simulink model "Xe_Model_Redo_June_26"  (R2018a)
settings: Solver=VariableStepAuto  StartTime=0.0  StopTime=5E5+96*60*60  RelTol=1e-3
values from neighbouring files (symbols this model uses):
  A_pipe = pi*r_pipe^2    (= 0.0126676869774)    [Startup_Script.m]
  alpha_FS = 0.517E-16    (= 5.17e-17)    [Startup_Script.m]
  alpha_G_R1 = 0.334E-17    (= 3.34e-18)    [Startup_Script.m]
  alpha_G_R2 = 0.699E-17    (= 6.99e-18)    [Startup_Script.m]
  alpha_G_R3 = 0.669E-17    (= 6.69e-18)    [Startup_Script.m]
  alpha_G_R4 = 0.791E-18    (= 7.91e-19)    [Startup_Script.m]
  D_g = 2.37E-9    (= 2.37e-09)    [Startup_Script.m]
  epsilon = 0.1    [Startup_Script.m]
  eta_b = 1E-4    (= 0.0001)    [Startup_Script.m]
  eta_fs = 1.2E-4    (= 0.00012)    [Startup_Script.m]
  f_cv = 0.004    [Startup_Script.m]
  FS_Mu_A = 4340    [Startup_Script.m]
  FS_Mu_K = 0.084    [Startup_Script.m]
  FS_Mu_MSRE = 0.007027    [Startup_Script.m]
  FS_rho_A = 3.628    [Startup_Script.m]
  FS_rho_B = 0.00066    [Startup_Script.m]
  FS_rho_MSRE = 2082    [Startup_Script.m]
  gamma_i = 0.0293524    [Startup_Script.m]
  gamma_te = 0.0322482    [Startup_Script.m]
  gamma_xe = 0.00257324    [Startup_Script.m]
  h_fc = 1.6    [Startup_Script.m]
  H_Xe_a = 5.713e-13    [Startup_Script.m]
  H_Xe_b = -7.937e-10    [Startup_Script.m]
  H_Xe_c = 2.809e-07    [Startup_Script.m]
  HX_r_Tube = ((0.5-0.042)/2)*2.54E-2    (= 0.0058166)    [Startup_Script.m]
  HX_XS = HX_N_Tubes*(pi*HX_r_Tube^2)    (= 0.0168999490356)    [Startup_Script.m]
  k_b = 1.3806E-23    (= 1.3806e-23)    [Startup_Script.m]
  lambda_i = 2.9306070546251702E-5    (= 2.93060705463e-05)    [Startup_Script.m]
  lambda_te = 0.036481430555786593    (= 0.0364814305558)    [Startup_Script.m]
  lambda_xe = 2.0924e-05    [Startup_Script.m]
  N_FC_R1 = 12    [Startup_Script.m]
  N_FC_R2 = 940    [Startup_Script.m]
  N_FC_R3 = 108    [Startup_Script.m]
  N_FC_R4 = 78    [Startup_Script.m]
  P_pump = 35420    [Startup_Script.m]
  phi0 = 3.98E+17    (= 3.98e+17)    [Startup_Script.m]
  phi_G_R_1 = mean(interp1(phi_G_R,phi_G_phi, linspace(0,r_g_r1)))    [Startup_Script.m]
  phi_G_R_2 = mean(interp1(phi_G_R,phi_G_phi, linspace(r_g_r1,r_g_r2)))    [Startup_Script.m]
  phi_G_R_3 = mean(interp1(phi_G_R,phi_G_phi, linspace(r_g_r2,r_g_r3)))    [Startup_Script.m]
  phi_G_R_4 = mean(interp1(phi_G_R,phi_G_phi, linspace(r_g_r3,r_g_r4)))    [Startup_Script.m]
  Q_strpr = 0.003155    [Startup_Script.m]
  Q_tot = 0.07571    [Startup_Script.m]
  r_b = 0.000254    [Startup_Script.m]
  r_fc = 0.79e-2    (= 0.0079)    [Startup_Script.m]
  r_pipe = (5E-2*2.54)/2    (= 0.0635)    [Startup_Script.m]
  r_xe = 2.16E-10    (= 2.16e-10)    [Startup_Script.m]
  Re_CA = 25800    [Startup_Script.m]
  Re_LH = 1E4    (= 10000)    [Startup_Script.m]
  Re_UH = 1E4    (= 10000)    [Startup_Script.m]
  sig_a_xe = 1.18E-22    (= 1.18e-22)    [Startup_Script.m]
  Sig_f = 0.15    [Startup_Script.m]
  T_CA_0 = T_INLET    (= 907.594444444)    [Startup_Script.m]
  T_FP_0 = T_OUTLET    (= 935.372222222)    [Startup_Script.m]
  T_FS_R_1_0 = mean(interp1(R_fs_m,T_fs_K, linspace(0,r_g_r1)))    [Startup_Script.m]
  T_FS_R_2_0 = mean(interp1(R_fs_m,T_fs_K, linspace(r_g_r1,r_g_r2)))    [Startup_Script.m]
  T_FS_R_3_0 = mean(interp1(R_fs_m,T_fs_K, linspace(r_g_r2,r_g_r3)))    [Startup_Script.m]
  T_FS_R_4_0 = mean(interp1(R_fs_m,T_fs_K, linspace(r_g_r3,r_g_r4)))    [Startup_Script.m]
  T_G_R_1_0 = mean(interp1(R_gr_m,T_gr_K, linspace(0,r_g_r1)))    [Startup_Script.m]
  T_HX_0 = 0.5*(T_OUTLET + T_INLET)    (= 921.483333333)    [Startup_Script.m]
  T_LH_0 = T_INLET    (= 907.594444444)    [Startup_Script.m]
  T_Mes = 928.15    [Startup_Script.m]
  T_P100_0 = T_OUTLET    (= 935.372222222)    [Startup_Script.m]
  T_P101_0 = T_OUTLET    (= 935.372222222)    [Startup_Script.m]
  T_P102_0 = T_INLET    (= 907.594444444)    [Startup_Script.m]
  T_Salt_0 = 900    [Startup_Script.m]
  T_UH_0 = T_OUTLET    (= 935.372222222)    [Startup_Script.m]
  U_FC_R1 = 0.607    [Startup_Script.m]
  U_FC_R2 = 0.183    [Startup_Script.m]
  U_FC_R3 = 0.454    [Startup_Script.m]
  U_FC_R4 = 0.250    (= 0.25)    [Startup_Script.m]
  V_CA_0 = 9.7*cubed_foot_to_cubed_meter    (= 0.274673445)    [Startup_Script.m]
  V_FP_0 = (0.9+3.2)*cubed_foot_to_cubed_meter    (= 0.116099085)    [Startup_Script.m]
  V_HX_0 = 6.1*cubed_foot_to_cubed_meter    (= 0.172732785)    [Startup_Script.m]
  V_LH_0 = 10.0*cubed_foot_to_cubed_meter    (= 0.2831685)    [Startup_Script.m]
  V_P100_0 = 2.1*cubed_foot_to_cubed_meter    (= 0.059465385)    [Startup_Script.m]
  V_P101_0 = 0.8*cubed_foot_to_cubed_meter    (= 0.02265348)    [Startup_Script.m]
  V_P102_0 = 2.2*cubed_foot_to_cubed_meter    (= 0.06229707)    [Startup_Script.m]
  V_R1_0 = V_Core_FS_0 *N_FC_R1/N_FC_tot    (= 0.00753107712766)    [Startup_Script.m]
  V_R2_0 = V_Core_FS_0 *N_FC_R2/N_FC_tot    (= 0.589934375)    [Startup_Script.m]
  V_R3_0 = V_Core_FS_0 *N_FC_R3/N_FC_tot    (= 0.0677796941489)    [Startup_Script.m]
  V_R4_0 = V_Core_FS_0 *N_FC_R4/N_FC_tot    (= 0.0489520013298)    [Startup_Script.m]
  V_UH_0 = 10.5*cubed_foot_to_cubed_meter    (= 0.297326925)    [Startup_Script.m]
undefined symbols (not defined in the file or in its folder): magnitude, V_CA, V_HX, V_P2, V_P3, V_R1, V_R2, V_R3, V_R4, V_UH
libraries: simulink x4, dspindex x4, dspstat3 x4, SignalEditorBlockLib x2
(part 5 of 11)

== system Xe_Model_Redo_June_26/Graphite /Graphite Region 4/Graphite Stringer/HMat ==
  H_Mat : Inport
  T : Inport  Port=2
  k_m_g : Inport  Port=3
  rGhost : Inport  Port=4
  Calc H_Xe : Subsystem
  H_Gain : Product  Inputs=****//
  mul : Product
  Out1 : Outport
  wires:
  H_Mat/1 -> mul/1
  mul/1 -> Out1/1
  H_Gain/1 -> mul/2
  rGhost/1 -> H_Gain/6
  Calc H_Xe/1(H_Xe [m^-3 Pa^-1]) -> H_Gain/1
  T/1 -> Calc H_Xe/1(T_Salt [K]), H_Gain/3
  k_m_g/1 -> H_Gain/4
  [epsilon] -> H_Gain/5
  [R_gas] -> H_Gain/2

== system Xe_Model_Redo_June_26/Bubbles/Bubble Mass Transfer/Bubble Total KMA/HX KMA/CA  CV Area ==
  Node Vol. : Inport
  Node T : Inport  Port=2
  CV Vol to Mass Transfer Area1 : Subsystem
  Calc CV Vol W Temp : Subsystem
  A : Outport
  wires:
  CV Vol to Mass Transfer Area1/1(A) -> A/1
  Node T/1 -> Calc CV Vol W Temp/2(T)
  Node Vol./1 -> Calc CV Vol W Temp/1(Vol. Gas)
  Calc CV Vol W Temp/1(V Gas) -> CV Vol to Mass Transfer Area1/1(V)

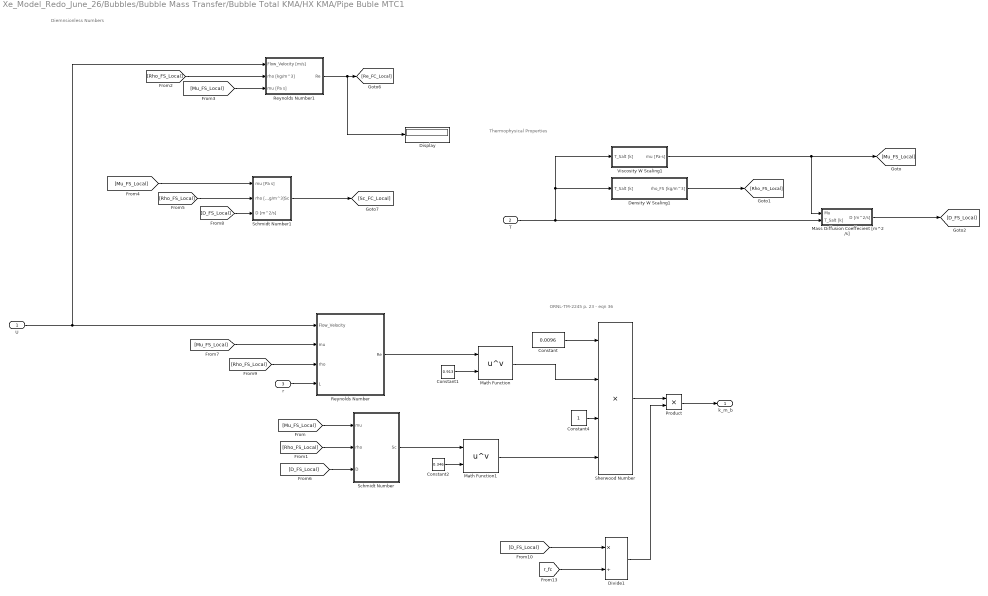
== system Xe_Model_Redo_June_26/Bubbles/Bubble Mass Transfer/Bubble Total KMA/HX KMA/Pipe Buble MTC1 ==
  note: ORNL-TM-2245 p. 23 - eqn 36
  note: Diemnsionless Numbers
  note: Thermophysical Properties
  U : Inport
  T : Inport  Port=2
  r : Inport  Port=3
  Constant : Constant  Value=0.0096
  Constant1 : Constant  Value=0.913
  Constant2 : Constant  Value=0.346
  Constant4 : Constant
  Density W Scaling1 : Subsystem
  Display : Display
  Divide1 : Product  Inputs=*/
  Mass Diffusion Coeffecient [m^2 /s] : Subsystem
  Math Function : Math  Operator=pow  SaturateOnIntegerOverflow=on
  Math Function1 : Math  Operator=pow  SaturateOnIntegerOverflow=on
  Product : Product
  Reynolds Number : Subsystem
  Reynolds Number1 : Subsystem
  Schmidt Number : Subsystem
  Schmidt Number1 : Subsystem
  Sherwood Number : Product  Inputs=4
  Viscosity W Scaling1 : Subsystem
  k_m_b : Outport
  wires:
  Constant1/1 -> Math Function/2
  [r_fc] -> Divide1/2
  Constant2/1 -> Math Function1/2
  [D_FS_Local] -> Divide1/1
  Constant4/1 -> Sherwood Number/3
  Constant/1 -> Sherwood Number/1
  Divide1/1 -> Product/2
  Math Function1/1 -> Sherwood Number/4
  Schmidt Number/1(Sc) -> Math Function1/1
  Math Function/1 -> Sherwood Number/2
  Sherwood Number/1 -> Product/1
  Product/1 -> k_m_b/1
  Reynolds Number/1(Re) -> Math Function/1
  Schmidt Number1/1(Sc) -> [Sc_FC_Local]
  Reynolds Number1/1(Re) -> Display/1, [Re_FC_Local]
  U/1 -> Reynolds Number1/1(Flow_Velocity [m/s]), Reynolds Number/1(Flow_Velocity)
  [Rho_FS_Local] -> Reynolds Number1/2(rho [kg/m^3])
  [Mu_FS_Local] -> Reynolds Number1/3(mu [Pa s])
  [Mu_FS_Local] -> Schmidt Number1/1(mu [Pa s])
  [Rho_FS_Local] -> Schmidt Number1/2(rho [kg/m^3])
  [D_FS_Local] -> Schmidt Number1/3(D [m^2/s])
  [Mu_FS_Local] -> Schmidt Number/1(mu)
  [Rho_FS_Local] -> Schmidt Number/2(rho)
  [D_FS_Local] -> Schmidt Number/3(D)
  [Mu_FS_Local] -> Reynolds Number/2(mu)
  [Rho_FS_Local] -> Reynolds Number/3(rho)
  r/1 -> Reynolds Number/4(L)
  T/1 -> Mass Diffusion Coeffecient [m^2 /s]/2(T_Salt [k]), Viscosity W Scaling1/1(T_Salt [k]), Density W Scaling1/1(T_Salt [k])
  Density W Scaling1/1(rho_FS [kg/m^3]) -> [Rho_FS_Local]
  Viscosity W Scaling1/1(mu [Pa-s]) -> Mass Diffusion Coeffecient [m^2 /s]/1(Mu), [Mu_FS_Local]
  Mass Diffusion Coeffecient [m^2 /s]/1(D [m^2/s]) -> [D_FS_Local]

== system Xe_Model_Redo_June_26/Bubbles/Bubble Mass Transfer/Bubble Total KMA/KMA FP/CA  CV Area ==
  Node Vol. : Inport
  Node T : Inport  Port=2
  CV Vol to Mass Transfer Area1 : Subsystem
  Calc CV Vol W Temp : Subsystem
  A : Outport
  wires:
  CV Vol to Mass Transfer Area1/1(A) -> A/1
  Node T/1 -> Calc CV Vol W Temp/2(T)
  Node Vol./1 -> Calc CV Vol W Temp/1(Vol. Gas)
  Calc CV Vol W Temp/1(V Gas) -> CV Vol to Mass Transfer Area1/1(V)

== system Xe_Model_Redo_June_26/Bubbles/Bubble Mass Transfer/Bubble Total KMA/KMA FP/Pump Bowl MTC1 ==
  note: Perry's 5-70
  note: Thermophysical Properties
  T : Inport
  Constant : Constant  Value=0.13
  Constant1 : Constant  Value=P_pump
  Constant3 : Constant  Value=1/4
  Constant4 : Constant  Value=2/3
  Density W Scaling1 : Subsystem
  Divide : Product  Inputs=*/
  Divide1 : Product  Inputs=*/
  Divide2 : Product  Inputs=*/
  Mass Diffusion Coeffecient [m^2 /s] : Subsystem
  Math Function : Math  Operator=magnitude^2  SaturateOnIntegerOverflow=on
  Math Function1 : Math  Operator=pow  SaturateOnIntegerOverflow=on
  Math Function3 : Math  Operator=pow  SaturateOnIntegerOverflow=on
  Product : Product
  Product1 : Product  Inputs=***
  Schmidt Number1 : Subsystem
  Viscosity W Scaling1 : Subsystem
  g_c : Constant  Value=9.81
  k_m : Outport
  wires:
  Divide/1 -> Product1/1
  Constant/1 -> Product/1
  [VF_FP] -> Divide/2
  Schmidt Number1/1(Sc) -> [Sc_FC_Local]
  [Rho_FS_Local] -> Schmidt Number1/2(rho [kg/m^3])
  [Mu_FS_Local] -> Schmidt Number1/1(mu [Pa s])
  [D_FS_Local] -> Schmidt Number1/3(D [m^2/s])
  Constant1/1 -> Divide/1
  [Mu_FS_Local] -> Product1/2
  g_c/1 -> Product1/3
  [Rho_FS_Local] -> Math Function/1
  Product1/1 -> Divide1/1
  Math Function/1 -> Divide1/2
  Constant3/1 -> Math Function1/2
  Divide1/1 -> Math Function1/1
  Math Function1/1 -> Product/2
  Product/1 -> Divide2/1
  [Sc_FC_Local] -> Math Function3/1
  Constant4/1 -> Math Function3/2
  Math Function3/1 -> Divide2/2
  Divide2/1 -> k_m/1
  T/1 -> Mass Diffusion Coeffecient [m^2 /s]/2(T_Salt [k]), Viscosity W Scaling1/1(T_Salt [k]), Density W Scaling1/1(T_Salt [k])
  Density W Scaling1/1(rho_FS [kg/m^3]) -> [Rho_FS_Local]
  Viscosity W Scaling1/1(mu [Pa-s]) -> Mass Diffusion Coeffecient [m^2 /s]/1(Mu), [Mu_FS_Local]
  Mass Diffusion Coeffecient [m^2 /s]/1(D [m^2/s]) -> [D_FS_Local]

== system Xe_Model_Redo_June_26/Bubbles/Bubble Mass Transfer/Bubble Total KMA/KMA_CA/CA  CV Area ==
  Node Vol. : Inport
  Node T : Inport  Port=2
  CV Vol to Mass Transfer Area1 : Subsystem
  Calc CV Vol W Temp : Subsystem
  A : Outport
  wires:
  CV Vol to Mass Transfer Area1/1(A) -> A/1
  Node T/1 -> Calc CV Vol W Temp/2(T)
  Node Vol./1 -> Calc CV Vol W Temp/1(Vol. Gas)
  Calc CV Vol W Temp/1(V Gas) -> CV Vol to Mass Transfer Area1/1(V)

== system Xe_Model_Redo_June_26/Bubbles/Bubble Mass Transfer/Bubble Total KMA/KMA_CA/CA  MTC ==
  note: Perry's P. 5-69
  note: Thermophysical Properties
  T : Inport
  Constant : Constant  Value=1.13
  Constant1 : Constant  Value=0.5
  Constant2 : Constant  Value=0.5
  Constant3 : Constant  Value=Re_CA
  Constant4 : Constant
  Density W Scaling1 : Subsystem
  Divide1 : Product  Inputs=*/
  Mass Diffusion Coeffecient [m^2 /s] : Subsystem
  Math Function : Math  Operator=pow  SaturateOnIntegerOverflow=on
  Math Function1 : Math  Operator=pow  SaturateOnIntegerOverflow=on
  Product : Product
  Re_Num  Scaled : Subsystem
  Schmidt Number : Subsystem
  Sherwood Number : Product  Inputs=4
  Viscosity W Scaling1 : Subsystem
  k_m_b : Outport
  wires:
  Constant1/1 -> Math Function/2
  [r_fc] -> Divide1/2
  Constant2/1 -> Math Function1/2
  [D_FS_Local] -> Divide1/1
  Constant4/1 -> Sherwood Number/3
  Constant/1 -> Sherwood Number/1
  Divide1/1 -> Product/2
  Math Function1/1 -> Sherwood Number/4
  Schmidt Number/1(Sc) -> Math Function1/1
  Math Function/1 -> Sherwood Number/2
  Sherwood Number/1 -> Product/1
  Product/1 -> k_m_b/1
  [Mu_FS_Local] -> Schmidt Number/1(mu)
  [Rho_FS_Local] -> Schmidt Number/2(rho)
  [D_FS_Local] -> Schmidt Number/3(D)
  Viscosity W Scaling1/1(mu [Pa-s]) -> Mass Diffusion Coeffecient [m^2 /s]/1(Mu), [Mu_FS_Local]
  Mass Diffusion Coeffecient [m^2 /s]/1(D [m^2/s]) -> [D_FS_Local]
  Density W Scaling1/1(rho_FS [kg/m^3]) -> [Rho_FS_Local]
  T/1 -> Re_Num  Scaled/1(T), Mass Diffusion Coeffecient [m^2 /s]/2(T_Salt [k]), Viscosity W Scaling1/1(T_Salt [k]), Density W Scaling1/1(T_Salt [k])
  Re_Num  Scaled/1(Re) -> Math Function/1
  Constant3/1 -> Re_Num  Scaled/2(Re_0)

== system Xe_Model_Redo_June_26/Bubbles/Bubble Mass Transfer/Bubble Total KMA/KMA_IC/R1 ==
  Constant : Constant  Value=V_R1
  P1 MTC : Subsystem
  R1  CV Area : Subsystem
  k_m A : Product
  kmA : Outport
  wires:
  [r_fc] -> P1 MTC/3(r)
  [U_FC_R1] -> P1 MTC/1(U)
  P1 MTC/1(k_m_b) -> k_m A/2
  k_m A/1 -> kmA/1
  Constant/1 -> R1  CV Area/1(Node Vol.)
  [T_G_R_1] -> R1  CV Area/2(Node T), P1 MTC/2(T)
  R1  CV Area/1(A) -> k_m A/1

== system Xe_Model_Redo_June_26/Bubbles/Bubble Mass Transfer/Bubble Total KMA/KMA_IC/R2 ==
  Constant : Constant  Value=V_R2
  P1 MTC : Subsystem
  R2  CV Area : Subsystem
  k_m A : Product
  kmA : Outport
  wires:
  [r_fc] -> P1 MTC/3(r)
  [U_FC_R2] -> P1 MTC/1(U)
  P1 MTC/1(k_m_b) -> k_m A/2
  k_m A/1 -> kmA/1
  Constant/1 -> R2  CV Area/1(Node Vol.)
  [T_G_R_2] -> R2  CV Area/2(Node T), P1 MTC/2(T)
  R2  CV Area/1(A) -> k_m A/1

== system Xe_Model_Redo_June_26/Bubbles/Bubble Mass Transfer/Bubble Total KMA/KMA_IC/R3 ==
  Constant : Constant  Value=V_R3
  P1 MTC : Subsystem
  R3  CV Area : Subsystem
  k_m A : Product
  kmA : Outport
  wires:
  [r_fc] -> P1 MTC/3(r)
  [U_FC_R3] -> P1 MTC/1(U)
  P1 MTC/1(k_m_b) -> k_m A/2
  k_m A/1 -> kmA/1
  Constant/1 -> R3  CV Area/1(Node Vol.)
  [T_G_R_3] -> R3  CV Area/2(Node T), P1 MTC/2(T)
  R3  CV Area/1(A) -> k_m A/1

== system Xe_Model_Redo_June_26/Bubbles/Bubble Mass Transfer/Bubble Total KMA/KMA_IC/R4 ==
  Constant : Constant  Value=V_R4
  P1 MTC : Subsystem
  R4  CV Area : Subsystem
  k_m A : Product
  kmA : Outport
  wires:
  [r_fc] -> P1 MTC/3(r)
  [U_FC_R4] -> P1 MTC/1(U)
  P1 MTC/1(k_m_b) -> k_m A/2
  k_m A/1 -> kmA/1
  Constant/1 -> R4  CV Area/1(Node Vol.)
  [T_G_R_4] -> R4  CV Area/2(Node T), P1 MTC/2(T)
  R4  CV Area/1(A) -> k_m A/1

== system Xe_Model_Redo_June_26/Bubbles/Bubble Mass Transfer/Bubble Total KMA/KMA_LH/LH  CV Area ==
  Node Vol. : Inport
  Node T : Inport  Port=2
  CV Vol to Mass Transfer Area1 : Subsystem
  Calc CV Vol W Temp : Subsystem
  A : Outport
  wires:
  CV Vol to Mass Transfer Area1/1(A) -> A/1
  Node T/1 -> Calc CV Vol W Temp/2(T)
  Node Vol./1 -> Calc CV Vol W Temp/1(Vol. Gas)
  Calc CV Vol W Temp/1(V Gas) -> CV Vol to Mass Transfer Area1/1(V)

== system Xe_Model_Redo_June_26/Bubbles/Bubble Mass Transfer/Bubble Total KMA/KMA_LH/MTC LH ==
  note: Perry's P. 5-69
  note: Diemnsionless Numbers
  note: Thermophysical Properties
  T : Inport
  Constant : Constant  Value=1.13
  Constant1 : Constant  Value=0.5
  Constant2 : Constant  Value=0.5
  Constant3 : Constant  Value=Re_LH
  Constant4 : Constant
  Density W Scaling1 : Subsystem
  Divide1 : Product  Inputs=*/
  Mass Diffusion Coeffecient [m^2 /s] : Subsystem
  Math Function : Math  Operator=pow  SaturateOnIntegerOverflow=on
  Math Function1 : Math  Operator=pow  SaturateOnIntegerOverflow=on
  Product : Product
  Re_Num  Scaled : Subsystem
  Schmidt Number : Subsystem
  Schmidt Number1 : Subsystem
  Sherwood Number : Product  Inputs=4
  Viscosity W Scaling1 : Subsystem
  k_m_b : Outport
  wires:
  Constant1/1 -> Math Function/2
  [r_fc] -> Divide1/2
  Constant2/1 -> Math Function1/2
  [D_FS_Local] -> Divide1/1
  Constant4/1 -> Sherwood Number/3
  Constant/1 -> Sherwood Number/1
  Divide1/1 -> Product/2
  Math Function1/1 -> Sherwood Number/4
  Schmidt Number/1(Sc) -> Math Function1/1
  Math Function/1 -> Sherwood Number/2
  Sherwood Number/1 -> Product/1
  Product/1 -> k_m_b/1
  Re_Num  Scaled/1(Re) -> Math Function/1
  Schmidt Number1/1(Sc) -> [Sc_FC_Local]
  [Mu_FS_Local] -> Schmidt Number1/1(mu [Pa s])
  [Rho_FS_Local] -> Schmidt Number1/2(rho [kg/m^3])
  [D_FS_Local] -> Schmidt Number1/3(D [m^2/s])
  [Mu_FS_Local] -> Schmidt Number/1(mu)
  [Rho_FS_Local] -> Schmidt Number/2(rho)
  [D_FS_Local] -> Schmidt Number/3(D)
  Density W Scaling1/1(rho_FS [kg/m^3]) -> [Rho_FS_Local]
  Viscosity W Scaling1/1(mu [Pa-s]) -> Mass Diffusion Coeffecient [m^2 /s]/1(Mu), [Mu_FS_Local]
  Mass Diffusion Coeffecient [m^2 /s]/1(D [m^2/s]) -> [D_FS_Local]
  Constant3/1 -> Re_Num  Scaled/2(Re_0)
  T/1 -> Re_Num  Scaled/1(T), Mass Diffusion Coeffecient [m^2 /s]/2(T_Salt [k]), Viscosity W Scaling1/1(T_Salt [k]), Density W Scaling1/1(T_Salt [k])

== system Xe_Model_Redo_June_26/Bubbles/Bubble Mass Transfer/Bubble Total KMA/KMA_UH/MTC UH ==
  note: Perry's P. 5-69
  note: Diemnsionless Numbers
  note: Thermophysical Properties
  T : Inport
  Constant : Constant  Value=1.13
  Constant1 : Constant  Value=0.5
  Constant2 : Constant  Value=0.5
  Constant3 : Constant  Value=Re_LH
  Constant4 : Constant
  Density W Scaling1 : Subsystem
  Divide1 : Product  Inputs=*/
  Mass Diffusion Coeffecient [m^2 /s]1 : Subsystem
  Math Function : Math  Operator=pow  SaturateOnIntegerOverflow=on
  Math Function1 : Math  Operator=pow  SaturateOnIntegerOverflow=on
  Product : Product
  Re_Num  Scaled : Subsystem
  Schmidt Number : Subsystem
  Schmidt Number1 : Subsystem
  Sherwood Number : Product  Inputs=4
  Viscosity W Scaling1 : Subsystem
  k_m_b : Outport
  wires:
  Constant1/1 -> Math Function/2
  [r_fc] -> Divide1/2
  Constant2/1 -> Math Function1/2
  [D_FS_Local] -> Divide1/1
  Constant4/1 -> Sherwood Number/3
  Constant/1 -> Sherwood Number/1
  Divide1/1 -> Product/2
  Math Function1/1 -> Sherwood Number/4
  Schmidt Number/1(Sc) -> Math Function1/1
  Math Function/1 -> Sherwood Number/2
  Sherwood Number/1 -> Product/1
  Product/1 -> k_m_b/1
  Re_Num  Scaled/1(Re) -> Math Function/1
  Schmidt Number1/1(Sc) -> [Sc_FC_Local]
  [Mu_FS_Local] -> Schmidt Number1/1(mu [Pa s])
  [Rho_FS_Local] -> Schmidt Number1/2(rho [kg/m^3])
  [D_FS_Local] -> Schmidt Number1/3(D [m^2/s])
  [Mu_FS_Local] -> Schmidt Number/1(mu)
  [Rho_FS_Local] -> Schmidt Number/2(rho)
  [D_FS_Local] -> Schmidt Number/3(D)
  T/1 -> Mass Diffusion Coeffecient [m^2 /s]1/2(T_Salt [k]), Viscosity W Scaling1/1(T_Salt [k]), Density W Scaling1/1(T_Salt [k]), Re_Num  Scaled/1(T)
  Density W Scaling1/1(rho_FS [kg/m^3]) -> [Rho_FS_Local]
  Viscosity W Scaling1/1(mu [Pa-s]) -> Mass Diffusion Coeffecient [m^2 /s]1/1(Mu), [Mu_FS_Local]
  Mass Diffusion Coeffecient [m^2 /s]1/1(D [m^2/s]) -> [D_FS_Local]
  Constant3/1 -> Re_Num  Scaled/2(Re_0)

== system Xe_Model_Redo_June_26/Bubbles/Bubble Mass Transfer/Bubble Total KMA/KMA_UH/UH CV Area ==
  Node Vol. : Inport
  Node T : Inport  Port=2
  CV Vol to Mass Transfer Area1 : Subsystem
  Calc CV Vol W Temp : Subsystem
  A : Outport
  wires:
  CV Vol to Mass Transfer Area1/1(A) -> A/1
  Node T/1 -> Calc CV Vol W Temp/2(T)
  Node Vol./1 -> Calc CV Vol W Temp/1(Vol. Gas)
  Calc CV Vol W Temp/1(V Gas) -> CV Vol to Mass Transfer Area1/1(V)

== system Xe_Model_Redo_June_26/Bubbles/Bubble Mass Transfer/Bubble Total KMA/P1 KMA/CA  CV Area ==
  Node Vol. : Inport
  Node T : Inport  Port=2
  CV Vol to Mass Transfer Area1 : Subsystem
  Calc CV Vol W Temp : Subsystem
  A : Outport
  wires:
  CV Vol to Mass Transfer Area1/1(A) -> A/1
  Node T/1 -> Calc CV Vol W Temp/2(T)
  Node Vol./1 -> Calc CV Vol W Temp/1(Vol. Gas)
  Calc CV Vol W Temp/1(V Gas) -> CV Vol to Mass Transfer Area1/1(V)

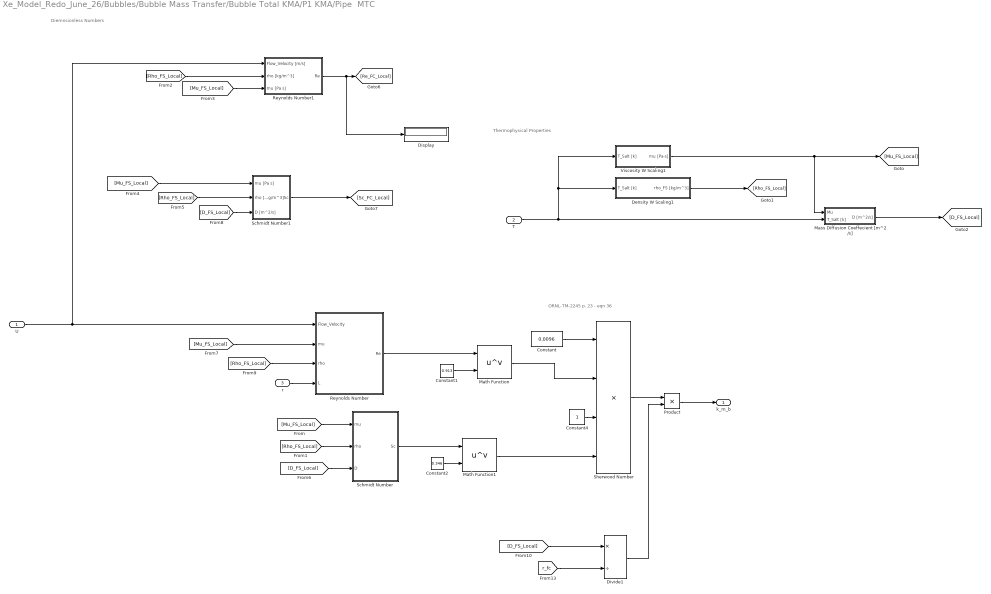
== system Xe_Model_Redo_June_26/Bubbles/Bubble Mass Transfer/Bubble Total KMA/P1 KMA/Pipe  MTC ==
  note: ORNL-TM-2245 p. 23 - eqn 36
  note: Diemnsionless Numbers
  note: Thermophysical Properties
  U : Inport
  T : Inport  Port=2
  r : Inport  Port=3
  Constant : Constant  Value=0.0096
  Constant1 : Constant  Value=0.913
  Constant2 : Constant  Value=0.346
  Constant4 : Constant
  Density W Scaling1 : Subsystem
  Display : Display
  Divide1 : Product  Inputs=*/
  Mass Diffusion Coeffecient [m^2 /s] : Subsystem
  Math Function : Math  Operator=pow  SaturateOnIntegerOverflow=on
  Math Function1 : Math  Operator=pow  SaturateOnIntegerOverflow=on
  Product : Product
  Reynolds Number : Subsystem
  Reynolds Number1 : Subsystem
  Schmidt Number : Subsystem
  Schmidt Number1 : Subsystem
  Sherwood Number : Product  Inputs=4
  Viscosity W Scaling1 : Subsystem
  k_m_b : Outport
  wires:
  Constant1/1 -> Math Function/2
  [r_fc] -> Divide1/2
  Constant2/1 -> Math Function1/2
  [D_FS_Local] -> Divide1/1
  Constant4/1 -> Sherwood Number/3
  Constant/1 -> Sherwood Number/1
  Divide1/1 -> Product/2
  Math Function1/1 -> Sherwood Number/4
  Schmidt Number/1(Sc) -> Math Function1/1
  Math Function/1 -> Sherwood Number/2
  Sherwood Number/1 -> Product/1
  Product/1 -> k_m_b/1
  Reynolds Number/1(Re) -> Math Function/1
  Schmidt Number1/1(Sc) -> [Sc_FC_Local]
  Reynolds Number1/1(Re) -> Display/1, [Re_FC_Local]
  U/1 -> Reynolds Number1/1(Flow_Velocity [m/s]), Reynolds Number/1(Flow_Velocity)
  [Rho_FS_Local] -> Reynolds Number1/2(rho [kg/m^3])
  [Mu_FS_Local] -> Reynolds Number1/3(mu [Pa s])
  [Mu_FS_Local] -> Schmidt Number1/1(mu [Pa s])
  [Rho_FS_Local] -> Schmidt Number1/2(rho [kg/m^3])
  [D_FS_Local] -> Schmidt Number1/3(D [m^2/s])
  [Mu_FS_Local] -> Schmidt Number/1(mu)
  [Rho_FS_Local] -> Schmidt Number/2(rho)
  [D_FS_Local] -> Schmidt Number/3(D)
  [Mu_FS_Local] -> Reynolds Number/2(mu)
  [Rho_FS_Local] -> Reynolds Number/3(rho)
  r/1 -> Reynolds Number/4(L)
  T/1 -> Mass Diffusion Coeffecient [m^2 /s]/2(T_Salt [k]), Viscosity W Scaling1/1(T_Salt [k]), Density W Scaling1/1(T_Salt [k])
  Density W Scaling1/1(rho_FS [kg/m^3]) -> [Rho_FS_Local]
  Viscosity W Scaling1/1(mu [Pa-s]) -> Mass Diffusion Coeffecient [m^2 /s]/1(Mu), [Mu_FS_Local]
  Mass Diffusion Coeffecient [m^2 /s]/1(D [m^2/s]) -> [D_FS_Local]

== system Xe_Model_Redo_June_26/Bubbles/Bubble Mass Transfer/Bubble Total KMA/P2 KMA/P2  CV Area ==
  Node Vol. : Inport
  Node T : Inport  Port=2
  CV Vol to Mass Transfer Area1 : Subsystem
  Calc CV Vol W Temp : Subsystem
  A : Outport
  wires:
  CV Vol to Mass Transfer Area1/1(A) -> A/1
  Node T/1 -> Calc CV Vol W Temp/2(T)
  Node Vol./1 -> Calc CV Vol W Temp/1(Vol. Gas)
  Calc CV Vol W Temp/1(V Gas) -> CV Vol to Mass Transfer Area1/1(V)

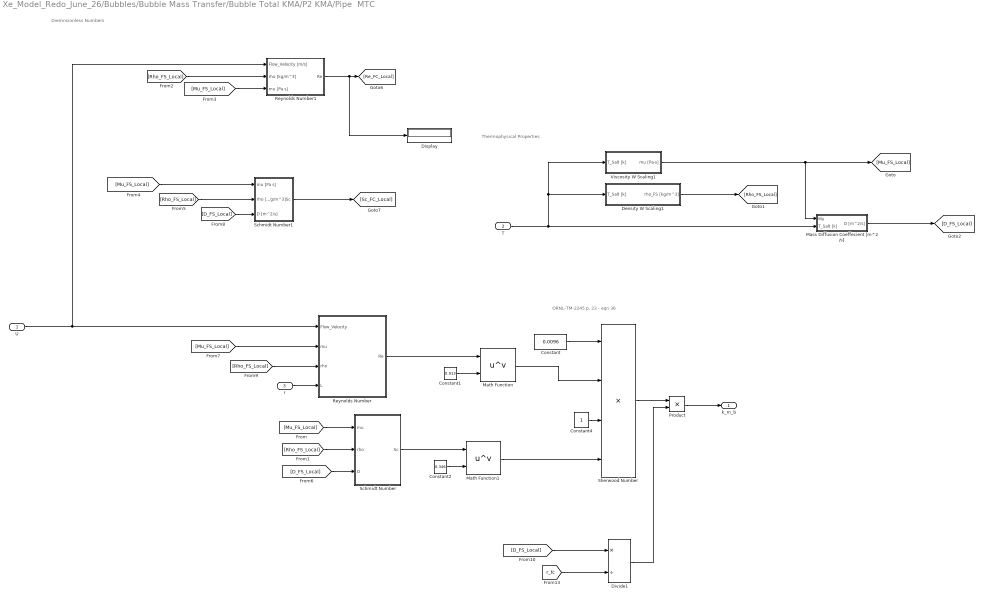
== system Xe_Model_Redo_June_26/Bubbles/Bubble Mass Transfer/Bubble Total KMA/P2 KMA/Pipe  MTC ==
  note: ORNL-TM-2245 p. 23 - eqn 36
  note: Diemnsionless Numbers
  note: Thermophysical Properties
  U : Inport
  T : Inport  Port=2
  r : Inport  Port=3
  Constant : Constant  Value=0.0096
  Constant1 : Constant  Value=0.913
  Constant2 : Constant  Value=0.346
  Constant4 : Constant
  Density W Scaling1 : Subsystem
  Display : Display
  Divide1 : Product  Inputs=*/
  Mass Diffusion Coeffecient [m^2 /s] : Subsystem
  Math Function : Math  Operator=pow  SaturateOnIntegerOverflow=on
  Math Function1 : Math  Operator=pow  SaturateOnIntegerOverflow=on
  Product : Product
  Reynolds Number : Subsystem
  Reynolds Number1 : Subsystem
  Schmidt Number : Subsystem
  Schmidt Number1 : Subsystem
  Sherwood Number : Product  Inputs=4
  Viscosity W Scaling1 : Subsystem
  k_m_b : Outport
  wires:
  Constant1/1 -> Math Function/2
  [r_fc] -> Divide1/2
  Constant2/1 -> Math Function1/2
  [D_FS_Local] -> Divide1/1
  Constant4/1 -> Sherwood Number/3
  Constant/1 -> Sherwood Number/1
  Divide1/1 -> Product/2
  Math Function1/1 -> Sherwood Number/4
  Schmidt Number/1(Sc) -> Math Function1/1
  Math Function/1 -> Sherwood Number/2
  Sherwood Number/1 -> Product/1
  Product/1 -> k_m_b/1
  Reynolds Number/1(Re) -> Math Function/1
  Schmidt Number1/1(Sc) -> [Sc_FC_Local]
  Reynolds Number1/1(Re) -> Display/1, [Re_FC_Local]
  U/1 -> Reynolds Number1/1(Flow_Velocity [m/s]), Reynolds Number/1(Flow_Velocity)
  [Rho_FS_Local] -> Reynolds Number1/2(rho [kg/m^3])
  [Mu_FS_Local] -> Reynolds Number1/3(mu [Pa s])
  [Mu_FS_Local] -> Schmidt Number1/1(mu [Pa s])
  [Rho_FS_Local] -> Schmidt Number1/2(rho [kg/m^3])
  [D_FS_Local] -> Schmidt Number1/3(D [m^2/s])
  [Mu_FS_Local] -> Schmidt Number/1(mu)
  [Rho_FS_Local] -> Schmidt Number/2(rho)
  [D_FS_Local] -> Schmidt Number/3(D)
  [Mu_FS_Local] -> Reynolds Number/2(mu)
  [Rho_FS_Local] -> Reynolds Number/3(rho)
  r/1 -> Reynolds Number/4(L)
  T/1 -> Mass Diffusion Coeffecient [m^2 /s]/2(T_Salt [k]), Viscosity W Scaling1/1(T_Salt [k]), Density W Scaling1/1(T_Salt [k])
  Density W Scaling1/1(rho_FS [kg/m^3]) -> [Rho_FS_Local]
  Viscosity W Scaling1/1(mu [Pa-s]) -> Mass Diffusion Coeffecient [m^2 /s]/1(Mu), [Mu_FS_Local]
  Mass Diffusion Coeffecient [m^2 /s]/1(D [m^2/s]) -> [D_FS_Local]

== system Xe_Model_Redo_June_26/Bubbles/Bubble Mass Transfer/Bubble Total KMA/P3 KMA/CA  CV Area ==
  Node Vol. : Inport
  Node T : Inport  Port=2
  CV Vol to Mass Transfer Area1 : Subsystem
  Calc CV Vol W Temp : Subsystem
  A : Outport
  wires:
  CV Vol to Mass Transfer Area1/1(A) -> A/1
  Node T/1 -> Calc CV Vol W Temp/2(T)
  Node Vol./1 -> Calc CV Vol W Temp/1(Vol. Gas)
  Calc CV Vol W Temp/1(V Gas) -> CV Vol to Mass Transfer Area1/1(V)

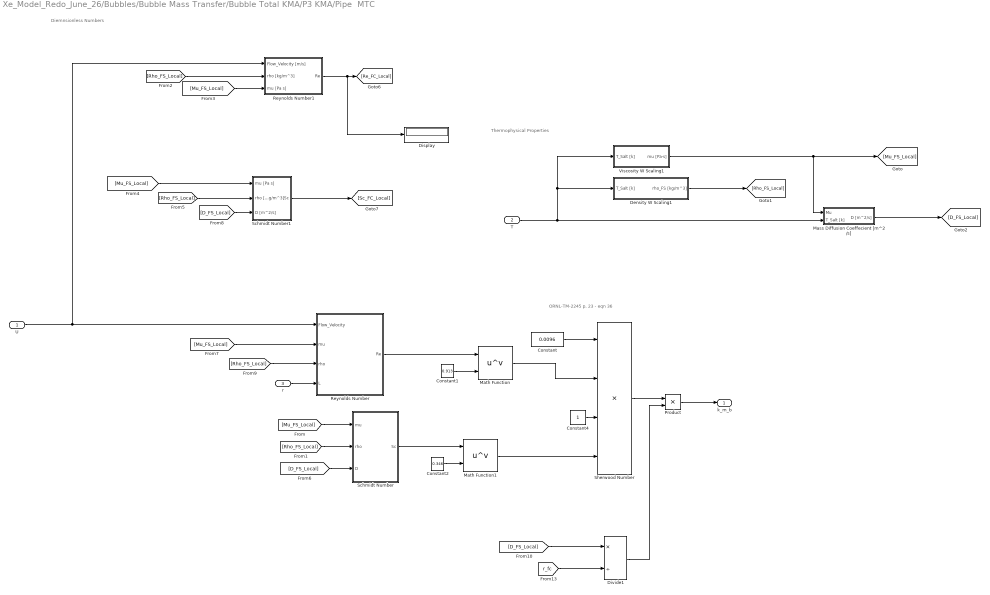
== system Xe_Model_Redo_June_26/Bubbles/Bubble Mass Transfer/Bubble Total KMA/P3 KMA/Pipe  MTC ==
  note: ORNL-TM-2245 p. 23 - eqn 36
  note: Diemnsionless Numbers
  note: Thermophysical Properties
  U : Inport
  T : Inport  Port=2
  r : Inport  Port=3
  Constant : Constant  Value=0.0096
  Constant1 : Constant  Value=0.913
  Constant2 : Constant  Value=0.346
  Constant4 : Constant
  Density W Scaling1 : Subsystem
  Display : Display
  Divide1 : Product  Inputs=*/
  Mass Diffusion Coeffecient [m^2 /s] : Subsystem
  Math Function : Math  Operator=pow  SaturateOnIntegerOverflow=on
  Math Function1 : Math  Operator=pow  SaturateOnIntegerOverflow=on
  Product : Product
  Reynolds Number : Subsystem
  Reynolds Number1 : Subsystem
  Schmidt Number : Subsystem
  Schmidt Number1 : Subsystem
  Sherwood Number : Product  Inputs=4
  Viscosity W Scaling1 : Subsystem
  k_m_b : Outport
  wires:
  Constant1/1 -> Math Function/2
  [r_fc] -> Divide1/2
  Constant2/1 -> Math Function1/2
  [D_FS_Local] -> Divide1/1
  Constant4/1 -> Sherwood Number/3
  Constant/1 -> Sherwood Number/1
  Divide1/1 -> Product/2
  Math Function1/1 -> Sherwood Number/4
  Schmidt Number/1(Sc) -> Math Function1/1
  Math Function/1 -> Sherwood Number/2
  Sherwood Number/1 -> Product/1
  Product/1 -> k_m_b/1
  Reynolds Number/1(Re) -> Math Function/1
  Schmidt Number1/1(Sc) -> [Sc_FC_Local]
  Reynolds Number1/1(Re) -> Display/1, [Re_FC_Local]
  U/1 -> Reynolds Number1/1(Flow_Velocity [m/s]), Reynolds Number/1(Flow_Velocity)
  [Rho_FS_Local] -> Reynolds Number1/2(rho [kg/m^3])
  [Mu_FS_Local] -> Reynolds Number1/3(mu [Pa s])
  [Mu_FS_Local] -> Schmidt Number1/1(mu [Pa s])
  [Rho_FS_Local] -> Schmidt Number1/2(rho [kg/m^3])
  [D_FS_Local] -> Schmidt Number1/3(D [m^2/s])
  [Mu_FS_Local] -> Schmidt Number/1(mu)
  [Rho_FS_Local] -> Schmidt Number/2(rho)
  [D_FS_Local] -> Schmidt Number/3(D)
  [Mu_FS_Local] -> Reynolds Number/2(mu)
  [Rho_FS_Local] -> Reynolds Number/3(rho)
  r/1 -> Reynolds Number/4(L)
  T/1 -> Mass Diffusion Coeffecient [m^2 /s]/2(T_Salt [k]), Viscosity W Scaling1/1(T_Salt [k]), Density W Scaling1/1(T_Salt [k])
  Density W Scaling1/1(rho_FS [kg/m^3]) -> [Rho_FS_Local]
  Viscosity W Scaling1/1(mu [Pa-s]) -> Mass Diffusion Coeffecient [m^2 /s]/1(Mu), [Mu_FS_Local]
  Mass Diffusion Coeffecient [m^2 /s]/1(D [m^2/s]) -> [D_FS_Local]

== system Xe_Model_Redo_June_26/Bubbles/Bubble Mass Transfer/CA/HRT*C_B /Calc H_Xe ==
  T_Salt [K] : Inport
  Constant : Constant  Value=H_Xe_c
  Math Function : Math  Operator=magnitude^2  SaturateOnIntegerOverflow=on
  Sum1 : Sum  Inputs=+++
  a const : Gain  Gain=H_Xe_a
  b const : Gain  Gain=H_Xe_b
  H_Xe [m^-3 Pa^-1] : Outport
  wires:
  Sum1/1 -> H_Xe [m^-3 Pa^-1]/1
  a const/1 -> Sum1/1
  Constant/1 -> Sum1/3
  b const/1 -> Sum1/2
  Math Function/1 -> a const/1
  T_Salt [K]/1 -> b const/1, Math Function/1

== system Xe_Model_Redo_June_26/Bubbles/Bubble Mass Transfer/CA/KMA_CA/CA  CV Area ==
  Node Vol. : Inport
  CV Vol to Mass Transfer Area1 : Subsystem
  A : Outport
  wires:
  CV Vol to Mass Transfer Area1/1(A) -> A/1
  Node Vol./1 -> CV Vol to Mass Transfer Area1/1(V)

== system Xe_Model_Redo_June_26/Bubbles/Bubble Mass Transfer/CA/KMA_CA/CA  MTC ==
  note: Perry's P. 5-69
  note: Thermophysical Properties
  T : Inport
  Constant : Constant  Value=1.0
  Constant1 : Constant  Value=1/3
  Constant2 : Constant  Value=1/3
  Constant3 : Constant  Value=Re_CA
  Constant4 : Constant
  Density W Scaling1 : Subsystem
  Divide1 : Product  Inputs=*/
  Gain : Gain  Gain=2
  Mass Diffusion Coeffecient [m^2 /s] : Subsystem
  Math Function : Math  Operator=pow  SaturateOnIntegerOverflow=on
  Math Function1 : Math  Operator=pow  SaturateOnIntegerOverflow=on
  Product : Product
  Re_Num  Scaled : Subsystem
  Schmidt Number : Subsystem
  Sherwood Number : Product  Inputs=4
  Viscosity W Scaling1 : Subsystem
  k_m_b : Outport
  wires:
  Constant1/1 -> Math Function/2
  Constant2/1 -> Math Function1/2
  [D_FS_Local] -> Divide1/1
  Constant4/1 -> Sherwood Number/3
  Constant/1 -> Sherwood Number/1
  Divide1/1 -> Product/2
  Math Function1/1 -> Sherwood Number/4
  Schmidt Number/1(Sc) -> Math Function1/1
  Math Function/1 -> Sherwood Number/2
  Sherwood Number/1 -> Product/1
  Product/1 -> k_m_b/1
  [Mu_FS_Local] -> Schmidt Number/1(mu)
  [Rho_FS_Local] -> Schmidt Number/2(rho)
  [D_FS_Local] -> Schmidt Number/3(D)
  Viscosity W Scaling1/1(mu [Pa-s]) -> Mass Diffusion Coeffecient [m^2 /s]/1(Mu), [Mu_FS_Local]
  Mass Diffusion Coeffecient [m^2 /s]/1(D [m^2/s]) -> [D_FS_Local]
  Density W Scaling1/1(rho_FS [kg/m^3]) -> [Rho_FS_Local]
  T/1 -> Re_Num  Scaled/1(T), Mass Diffusion Coeffecient [m^2 /s]/2(T_Salt [k]), Viscosity W Scaling1/1(T_Salt [k]), Density W Scaling1/1(T_Salt [k])
  Re_Num  Scaled/1(Re) -> Math Function/1
  Constant3/1 -> Re_Num  Scaled/2(Re_0)
  [r_b] -> Gain/1
  Gain/1 -> Divide1/2

== system Xe_Model_Redo_June_26/Bubbles/Bubble Mass Transfer/FP/HRT*C_B /Calc H_Xe ==
  T_Salt [K] : Inport
  Constant : Constant  Value=H_Xe_c
  Math Function : Math  Operator=magnitude^2  SaturateOnIntegerOverflow=on
  Sum1 : Sum  Inputs=+++
  a const : Gain  Gain=H_Xe_a
  b const : Gain  Gain=H_Xe_b
  H_Xe [m^-3 Pa^-1] : Outport
  wires:
  Sum1/1 -> H_Xe [m^-3 Pa^-1]/1
  a const/1 -> Sum1/1
  Constant/1 -> Sum1/3
  b const/1 -> Sum1/2
  Math Function/1 -> a const/1
  T_Salt [K]/1 -> b const/1, Math Function/1

== system Xe_Model_Redo_June_26/Bubbles/Bubble Mass Transfer/FP/KMA_FP/CA  CV Area ==
  Node Vol. : Inport
  CV Vol to Mass Transfer Area1 : Subsystem
  A : Outport
  wires:
  CV Vol to Mass Transfer Area1/1(A) -> A/1
  Node Vol./1 -> CV Vol to Mass Transfer Area1/1(V)

== system Xe_Model_Redo_June_26/Bubbles/Bubble Mass Transfer/FP/KMA_FP/Pump Bowl MTC ==
  note: Correlation 'G' Highly agitated systems; solid
      | particles, drops, and bubbles;
      | continuous phase coefficient
  note: Perry's 5-70
  note: Thermophysical Properties
  V_Node_Tot : Inport
  T : Inport  Port=2
  Constant : Constant  Value=0.13
  Constant1 : Constant  Value=P_pump
  Constant3 : Constant  Value=1/4
  Constant4 : Constant  Value=2/3
  Density W Scaling1 : Subsystem
  Divide : Product  Inputs=*/
  Divide1 : Product  Inputs=*/
  Divide2 : Product  Inputs=*/
  Mass Diffusion Coeffecient [m^2 /s] : Subsystem
  Math Function : Math  Operator=magnitude^2  SaturateOnIntegerOverflow=on
  Math Function1 : Math  Operator=pow  SaturateOnIntegerOverflow=on
  Math Function3 : Math  Operator=pow  SaturateOnIntegerOverflow=on
  Product : Product
  Product1 : Product  Inputs=***
  Schmidt Number1 : Subsystem
  Viscosity W Scaling1 : Subsystem
  g_c : Constant  Value=9.81
  k_m : Outport
  wires:
  Divide/1 -> Product1/1
  Constant/1 -> Product/1
  V_Node_Tot/1 -> Divide/2
  Schmidt Number1/1(Sc) -> [Sc_FC_Local]
  [Rho_FS_Local] -> Schmidt Number1/2(rho [kg/m^3])
  [Mu_FS_Local] -> Schmidt Number1/1(mu [Pa s])
  [D_FS_Local] -> Schmidt Number1/3(D [m^2/s])
  Constant1/1 -> Divide/1
  [Mu_FS_Local] -> Product1/2
  g_c/1 -> Product1/3
  [Rho_FS_Local] -> Math Function/1
  Product1/1 -> Divide1/1
  Math Function/1 -> Divide1/2
  Constant3/1 -> Math Function1/2
  Divide1/1 -> Math Function1/1
  Math Function1/1 -> Product/2
  Product/1 -> Divide2/1
  [Sc_FC_Local] -> Math Function3/1
  Constant4/1 -> Math Function3/2
  Math Function3/1 -> Divide2/2
  Divide2/1 -> k_m/1
  T/1 -> Mass Diffusion Coeffecient [m^2 /s]/2(T_Salt [k]), Viscosity W Scaling1/1(T_Salt [k]), Density W Scaling1/1(T_Salt [k])
  Density W Scaling1/1(rho_FS [kg/m^3]) -> [Rho_FS_Local]
  Viscosity W Scaling1/1(mu [Pa-s]) -> Mass Diffusion Coeffecient [m^2 /s]/1(Mu), [Mu_FS_Local]
  Mass Diffusion Coeffecient [m^2 /s]/1(D [m^2/s]) -> [D_FS_Local]

== system Xe_Model_Redo_June_26/Bubbles/Bubble Mass Transfer/G_R1/HRT*C_B /Calc H_Xe ==
  T_Salt [K] : Inport
  Constant : Constant  Value=H_Xe_c
  Math Function : Math  Operator=magnitude^2  SaturateOnIntegerOverflow=on
  Sum1 : Sum  Inputs=+++
  a const : Gain  Gain=H_Xe_a
  b const : Gain  Gain=H_Xe_b
  H_Xe [m^-3 Pa^-1] : Outport
  wires:
  Sum1/1 -> H_Xe [m^-3 Pa^-1]/1
  a const/1 -> Sum1/1
  Constant/1 -> Sum1/3
  b const/1 -> Sum1/2
  Math Function/1 -> a const/1
  T_Salt [K]/1 -> b const/1, Math Function/1

== system Xe_Model_Redo_June_26/Bubbles/Bubble Mass Transfer/G_R1/KMA_G_R1/CA  CV Area ==
  Node Vol. : Inport
  CV Vol to Mass Transfer Area1 : Subsystem
  A : Outport
  wires:
  CV Vol to Mass Transfer Area1/1(A) -> A/1
  Node Vol./1 -> CV Vol to Mass Transfer Area1/1(V)

== system Xe_Model_Redo_June_26/Bubbles/Bubble Mass Transfer/G_R1/KMA_G_R1/Pipe Bubble  MTC ==
  note: ORNL-TM-2245 p. 23 - eqn 36
  note: Thermophysical Properties
  U : Inport
  T : Inport  Port=2
  r : Inport  Port=3
  Constant : Constant  Value=0.0096
  Constant1 : Constant  Value=0.913
  Constant2 : Constant  Value=0.346
  Constant4 : Constant
  Density W Scaling1 : Subsystem
  Divide1 : Product  Inputs=*/
  Mass Diffusion Coeffecient [m^2 /s] : Subsystem
  Math Function : Math  Operator=pow  SaturateOnIntegerOverflow=on
  Math Function1 : Math  Operator=pow  SaturateOnIntegerOverflow=on
  Product : Product
  Reynolds Number : Subsystem
  Schmidt Number : Subsystem
  Sherwood Number : Product  Inputs=4
  Viscosity W Scaling1 : Subsystem
  k_m_b : Outport
  wires:
  Constant1/1 -> Math Function/2
  [r_fc] -> Divide1/2
  Constant2/1 -> Math Function1/2
  [D_FS_Local] -> Divide1/1
  Constant4/1 -> Sherwood Number/3
  Constant/1 -> Sherwood Number/1
  Divide1/1 -> Product/2
  Math Function1/1 -> Sherwood Number/4
  Schmidt Number/1(Sc) -> Math Function1/1
  Math Function/1 -> Sherwood Number/2
  Sherwood Number/1 -> Product/1
  Product/1 -> k_m_b/1
  Reynolds Number/1(Re) -> Math Function/1
  U/1 -> Reynolds Number/1(Flow_Velocity)
  [Mu_FS_Local] -> Schmidt Number/1(mu)
  [Rho_FS_Local] -> Schmidt Number/2(rho)
  [D_FS_Local] -> Schmidt Number/3(D)
  [Mu_FS_Local] -> Reynolds Number/2(mu)
  [Rho_FS_Local] -> Reynolds Number/3(rho)
  r/1 -> Reynolds Number/4(L)
  T/1 -> Mass Diffusion Coeffecient [m^2 /s]/2(T_Salt [k]), Viscosity W Scaling1/1(T_Salt [k]), Density W Scaling1/1(T_Salt [k])
  Density W Scaling1/1(rho_FS [kg/m^3]) -> [Rho_FS_Local]
  Viscosity W Scaling1/1(mu [Pa-s]) -> Mass Diffusion Coeffecient [m^2 /s]/1(Mu), [Mu_FS_Local]
  Mass Diffusion Coeffecient [m^2 /s]/1(D [m^2/s]) -> [D_FS_Local]

== system Xe_Model_Redo_June_26/Bubbles/Bubble Mass Transfer/G_R2/HRT*C_B /Calc H_Xe ==
  T_Salt [K] : Inport
  Constant : Constant  Value=H_Xe_c
  Math Function : Math  Operator=magnitude^2  SaturateOnIntegerOverflow=on
  Sum1 : Sum  Inputs=+++
  a const : Gain  Gain=H_Xe_a
  b const : Gain  Gain=H_Xe_b
  H_Xe [m^-3 Pa^-1] : Outport
  wires:
  Sum1/1 -> H_Xe [m^-3 Pa^-1]/1
  a const/1 -> Sum1/1
  Constant/1 -> Sum1/3
  b const/1 -> Sum1/2
  Math Function/1 -> a const/1
  T_Salt [K]/1 -> b const/1, Math Function/1

== system Xe_Model_Redo_June_26/Bubbles/Bubble Mass Transfer/G_R2/KMA_G_R1/CA  CV Area ==
  Node Vol. : Inport
  CV Vol to Mass Transfer Area1 : Subsystem
  A : Outport
  wires:
  CV Vol to Mass Transfer Area1/1(A) -> A/1
  Node Vol./1 -> CV Vol to Mass Transfer Area1/1(V)

== system Xe_Model_Redo_June_26/Bubbles/Bubble Mass Transfer/G_R2/KMA_G_R1/Pipe Bubble  MTC ==
  note: ORNL-TM-2245 p. 23 - eqn 36
  note: Thermophysical Properties
  U : Inport
  T : Inport  Port=2
  r : Inport  Port=3
  Constant : Constant  Value=0.0096
  Constant1 : Constant  Value=0.913
  Constant2 : Constant  Value=0.346
  Constant4 : Constant
  Density W Scaling1 : Subsystem
  Divide1 : Product  Inputs=*/
  Mass Diffusion Coeffecient [m^2 /s] : Subsystem
  Math Function : Math  Operator=pow  SaturateOnIntegerOverflow=on
  Math Function1 : Math  Operator=pow  SaturateOnIntegerOverflow=on
  Product : Product
  Reynolds Number : Subsystem
  Schmidt Number : Subsystem
  Sherwood Number : Product  Inputs=4
  Viscosity W Scaling1 : Subsystem
  k_m_b : Outport
  wires:
  Constant1/1 -> Math Function/2
  [r_fc] -> Divide1/2
  Constant2/1 -> Math Function1/2
  [D_FS_Local] -> Divide1/1
  Constant4/1 -> Sherwood Number/3
  Constant/1 -> Sherwood Number/1
  Divide1/1 -> Product/2
  Math Function1/1 -> Sherwood Number/4
  Schmidt Number/1(Sc) -> Math Function1/1
  Math Function/1 -> Sherwood Number/2
  Sherwood Number/1 -> Product/1
  Product/1 -> k_m_b/1
  Reynolds Number/1(Re) -> Math Function/1
  U/1 -> Reynolds Number/1(Flow_Velocity)
  [Mu_FS_Local] -> Schmidt Number/1(mu)
  [Rho_FS_Local] -> Schmidt Number/2(rho)
  [D_FS_Local] -> Schmidt Number/3(D)
  [Mu_FS_Local] -> Reynolds Number/2(mu)
  [Rho_FS_Local] -> Reynolds Number/3(rho)
  r/1 -> Reynolds Number/4(L)
  T/1 -> Mass Diffusion Coeffecient [m^2 /s]/2(T_Salt [k]), Viscosity W Scaling1/1(T_Salt [k]), Density W Scaling1/1(T_Salt [k])
  Density W Scaling1/1(rho_FS [kg/m^3]) -> [Rho_FS_Local]
  Viscosity W Scaling1/1(mu [Pa-s]) -> Mass Diffusion Coeffecient [m^2 /s]/1(Mu), [Mu_FS_Local]
  Mass Diffusion Coeffecient [m^2 /s]/1(D [m^2/s]) -> [D_FS_Local]

== system Xe_Model_Redo_June_26/Bubbles/Bubble Mass Transfer/G_R3/HRT*C_B /Calc H_Xe ==
  T_Salt [K] : Inport
  Constant : Constant  Value=H_Xe_c
  Math Function : Math  Operator=magnitude^2  SaturateOnIntegerOverflow=on
  Sum1 : Sum  Inputs=+++
  a const : Gain  Gain=H_Xe_a
  b const : Gain  Gain=H_Xe_b
  H_Xe [m^-3 Pa^-1] : Outport
  wires:
  Sum1/1 -> H_Xe [m^-3 Pa^-1]/1
  a const/1 -> Sum1/1
  Constant/1 -> Sum1/3
  b const/1 -> Sum1/2
  Math Function/1 -> a const/1
  T_Salt [K]/1 -> b const/1, Math Function/1

== system Xe_Model_Redo_June_26/Bubbles/Bubble Mass Transfer/G_R3/KMA_G_R1/CA  CV Area ==
  Node Vol. : Inport
  CV Vol to Mass Transfer Area1 : Subsystem
  A : Outport
  wires:
  CV Vol to Mass Transfer Area1/1(A) -> A/1
  Node Vol./1 -> CV Vol to Mass Transfer Area1/1(V)

== system Xe_Model_Redo_June_26/Bubbles/Bubble Mass Transfer/G_R3/KMA_G_R1/Pipe Bubble  MTC ==
  note: ORNL-TM-2245 p. 23 - eqn 36
  note: Thermophysical Properties
  U : Inport
  T : Inport  Port=2
  r : Inport  Port=3
  Constant : Constant  Value=0.0096
  Constant1 : Constant  Value=0.913
  Constant2 : Constant  Value=0.346
  Constant4 : Constant
  Density W Scaling1 : Subsystem
  Divide1 : Product  Inputs=*/
  Mass Diffusion Coeffecient [m^2 /s] : Subsystem
  Math Function : Math  Operator=pow  SaturateOnIntegerOverflow=on
  Math Function1 : Math  Operator=pow  SaturateOnIntegerOverflow=on
  Product : Product
  Reynolds Number : Subsystem
  Schmidt Number : Subsystem
  Sherwood Number : Product  Inputs=4
  Viscosity W Scaling1 : Subsystem
  k_m_b : Outport
  wires:
  Constant1/1 -> Math Function/2
  [r_fc] -> Divide1/2
  Constant2/1 -> Math Function1/2
  [D_FS_Local] -> Divide1/1
  Constant4/1 -> Sherwood Number/3
  Constant/1 -> Sherwood Number/1
  Divide1/1 -> Product/2
  Math Function1/1 -> Sherwood Number/4
  Schmidt Number/1(Sc) -> Math Function1/1
  Math Function/1 -> Sherwood Number/2
  Sherwood Number/1 -> Product/1
  Product/1 -> k_m_b/1
  Reynolds Number/1(Re) -> Math Function/1
  U/1 -> Reynolds Number/1(Flow_Velocity)
  [Mu_FS_Local] -> Schmidt Number/1(mu)
  [Rho_FS_Local] -> Schmidt Number/2(rho)
  [D_FS_Local] -> Schmidt Number/3(D)
  [Mu_FS_Local] -> Reynolds Number/2(mu)
  [Rho_FS_Local] -> Reynolds Number/3(rho)
  r/1 -> Reynolds Number/4(L)
  T/1 -> Mass Diffusion Coeffecient [m^2 /s]/2(T_Salt [k]), Viscosity W Scaling1/1(T_Salt [k]), Density W Scaling1/1(T_Salt [k])
  Density W Scaling1/1(rho_FS [kg/m^3]) -> [Rho_FS_Local]
  Viscosity W Scaling1/1(mu [Pa-s]) -> Mass Diffusion Coeffecient [m^2 /s]/1(Mu), [Mu_FS_Local]
  Mass Diffusion Coeffecient [m^2 /s]/1(D [m^2/s]) -> [D_FS_Local]

== system Xe_Model_Redo_June_26/Bubbles/Bubble Mass Transfer/G_R4/HRT*C_B /Calc H_Xe ==
  T_Salt [K] : Inport
  Constant : Constant  Value=H_Xe_c
  Math Function : Math  Operator=magnitude^2  SaturateOnIntegerOverflow=on
  Sum1 : Sum  Inputs=+++
  a const : Gain  Gain=H_Xe_a
  b const : Gain  Gain=H_Xe_b
  H_Xe [m^-3 Pa^-1] : Outport
  wires:
  Sum1/1 -> H_Xe [m^-3 Pa^-1]/1
  a const/1 -> Sum1/1
  Constant/1 -> Sum1/3
  b const/1 -> Sum1/2
  Math Function/1 -> a const/1
  T_Salt [K]/1 -> b const/1, Math Function/1

== system Xe_Model_Redo_June_26/Bubbles/Bubble Mass Transfer/G_R4/KMA_G_R1/CA  CV Area ==
  Node Vol. : Inport
  CV Vol to Mass Transfer Area1 : Subsystem
  A : Outport
  wires:
  CV Vol to Mass Transfer Area1/1(A) -> A/1
  Node Vol./1 -> CV Vol to Mass Transfer Area1/1(V)

== system Xe_Model_Redo_June_26/Bubbles/Bubble Mass Transfer/G_R4/KMA_G_R1/Pipe Bubble  MTC ==
  note: ORNL-TM-2245 p. 23 - eqn 36
  note: Thermophysical Properties
  U : Inport
  T : Inport  Port=2
  r : Inport  Port=3
  Constant : Constant  Value=0.0096
  Constant1 : Constant  Value=0.913
  Constant2 : Constant  Value=0.346
  Constant4 : Constant
  Density W Scaling1 : Subsystem
  Divide1 : Product  Inputs=*/
  Mass Diffusion Coeffecient [m^2 /s] : Subsystem
  Math Function : Math  Operator=pow  SaturateOnIntegerOverflow=on
  Math Function1 : Math  Operator=pow  SaturateOnIntegerOverflow=on
  Product : Product
  Reynolds Number : Subsystem
  Schmidt Number : Subsystem
  Sherwood Number : Product  Inputs=4
  Viscosity W Scaling1 : Subsystem
  k_m_b : Outport
  wires:
  Constant1/1 -> Math Function/2
  [r_fc] -> Divide1/2
  Constant2/1 -> Math Function1/2
  [D_FS_Local] -> Divide1/1
  Constant4/1 -> Sherwood Number/3
  Constant/1 -> Sherwood Number/1
  Divide1/1 -> Product/2
  Math Function1/1 -> Sherwood Number/4
  Schmidt Number/1(Sc) -> Math Function1/1
  Math Function/1 -> Sherwood Number/2
  Sherwood Number/1 -> Product/1
  Product/1 -> k_m_b/1
  Reynolds Number/1(Re) -> Math Function/1
  U/1 -> Reynolds Number/1(Flow_Velocity)
  [Mu_FS_Local] -> Schmidt Number/1(mu)
  [Rho_FS_Local] -> Schmidt Number/2(rho)
  [D_FS_Local] -> Schmidt Number/3(D)
  [Mu_FS_Local] -> Reynolds Number/2(mu)
  [Rho_FS_Local] -> Reynolds Number/3(rho)
  r/1 -> Reynolds Number/4(L)
  T/1 -> Mass Diffusion Coeffecient [m^2 /s]/2(T_Salt [k]), Viscosity W Scaling1/1(T_Salt [k]), Density W Scaling1/1(T_Salt [k])
  Density W Scaling1/1(rho_FS [kg/m^3]) -> [Rho_FS_Local]
  Viscosity W Scaling1/1(mu [Pa-s]) -> Mass Diffusion Coeffecient [m^2 /s]/1(Mu), [Mu_FS_Local]
  Mass Diffusion Coeffecient [m^2 /s]/1(D [m^2/s]) -> [D_FS_Local]

== system Xe_Model_Redo_June_26/Bubbles/Bubble Mass Transfer/HX/HRT*C_B /Calc H_Xe ==
  T_Salt [K] : Inport
  Constant : Constant  Value=H_Xe_c
  Math Function : Math  Operator=magnitude^2  SaturateOnIntegerOverflow=on
  Sum1 : Sum  Inputs=+++
  a const : Gain  Gain=H_Xe_a
  b const : Gain  Gain=H_Xe_b
  H_Xe [m^-3 Pa^-1] : Outport
  wires:
  Sum1/1 -> H_Xe [m^-3 Pa^-1]/1
  a const/1 -> Sum1/1
  Constant/1 -> Sum1/3
  b const/1 -> Sum1/2
  Math Function/1 -> a const/1
  T_Salt [K]/1 -> b const/1, Math Function/1

== system Xe_Model_Redo_June_26/Bubbles/Bubble Mass Transfer/HX/KMA_HX/CA  CV Area ==
  Node Vol. : Inport
  CV Vol to Mass Transfer Area1 : Subsystem
  A : Outport
  wires:
  CV Vol to Mass Transfer Area1/1(A) -> A/1
  Node Vol./1 -> CV Vol to Mass Transfer Area1/1(V)

== system Xe_Model_Redo_June_26/Bubbles/Bubble Mass Transfer/HX/KMA_HX/Pipe Buble MTC ==
  note: ORNL-TM-2245 p. 23 - eqn 36
  note: Thermophysical Properties
  U : Inport
  T : Inport  Port=2
  r : Inport  Port=3
  Constant : Constant  Value=0.0096
  Constant1 : Constant  Value=0.913
  Constant2 : Constant  Value=0.346
  Constant4 : Constant
  Density W Scaling1 : Subsystem
  Divide1 : Product  Inputs=*/
  Gain : Gain  Gain=2
  Mass Diffusion Coeffecient [m^2 /s] : Subsystem
  Math Function : Math  Operator=pow  SaturateOnIntegerOverflow=on
  Math Function1 : Math  Operator=pow  SaturateOnIntegerOverflow=on
  Product : Product
  Reynolds Number : Subsystem
  Schmidt Number : Subsystem
  Sherwood Number : Product  Inputs=4
  Viscosity W Scaling1 : Subsystem
  k_m_b : Outport
  wires:
  Constant1/1 -> Math Function/2
  r/1 -> Gain/1
  Constant2/1 -> Math Function1/2
  [D_FS_Local] -> Divide1/1
  Constant4/1 -> Sherwood Number/3
  Constant/1 -> Sherwood Number/1
  Divide1/1 -> Product/2
  Math Function1/1 -> Sherwood Number/4
  Schmidt Number/1(Sc) -> Math Function1/1
  Math Function/1 -> Sherwood Number/2
  Sherwood Number/1 -> Product/1
  Product/1 -> k_m_b/1
  Reynolds Number/1(Re) -> Math Function/1
  U/1 -> Reynolds Number/1(Flow_Velocity)
  [Mu_FS_Local] -> Schmidt Number/1(mu)
  [Rho_FS_Local] -> Schmidt Number/2(rho)
  [D_FS_Local] -> Schmidt Number/3(D)
  [Mu_FS_Local] -> Reynolds Number/2(mu)
  [Rho_FS_Local] -> Reynolds Number/3(rho)
  T/1 -> Mass Diffusion Coeffecient [m^2 /s]/2(T_Salt [k]), Viscosity W Scaling1/1(T_Salt [k]), Density W Scaling1/1(T_Salt [k])
  Density W Scaling1/1(rho_FS [kg/m^3]) -> [Rho_FS_Local]
  Viscosity W Scaling1/1(mu [Pa-s]) -> Mass Diffusion Coeffecient [m^2 /s]/1(Mu), [Mu_FS_Local]
  Mass Diffusion Coeffecient [m^2 /s]/1(D [m^2/s]) -> [D_FS_Local]
  Gain/1 -> Divide1/2, Reynolds Number/4(L)

== system Xe_Model_Redo_June_26/Bubbles/Bubble Mass Transfer/LH/HRT*C_B /Calc H_Xe ==
  T_Salt [K] : Inport
  Constant : Constant  Value=H_Xe_c
  Math Function : Math  Operator=magnitude^2  SaturateOnIntegerOverflow=on
  Sum1 : Sum  Inputs=+++
  a const : Gain  Gain=H_Xe_a
  b const : Gain  Gain=H_Xe_b
  H_Xe [m^-3 Pa^-1] : Outport
  wires:
  Sum1/1 -> H_Xe [m^-3 Pa^-1]/1
  a const/1 -> Sum1/1
  Constant/1 -> Sum1/3
  b const/1 -> Sum1/2
  Math Function/1 -> a const/1
  T_Salt [K]/1 -> b const/1, Math Function/1

== system Xe_Model_Redo_June_26/Bubbles/Bubble Mass Transfer/LH/KMA_LH/CA  CV Area ==
  Node Vol. : Inport
  CV Vol to Mass Transfer Area1 : Subsystem
  A : Outport
  wires:
  CV Vol to Mass Transfer Area1/1(A) -> A/1
  Node Vol./1 -> CV Vol to Mass Transfer Area1/1(V)

== system Xe_Model_Redo_June_26/Bubbles/Bubble Mass Transfer/LH/KMA_LH/MTC LH ==
  note: Perry's P. 5-69
  note: Thermophysical Properties
  T : Inport
  Constant : Constant  Value=1.0
  Constant1 : Constant  Value=1/3
  Constant2 : Constant  Value=1/3
  Constant3 : Constant  Value=Re_LH
  Constant4 : Constant
  Density W Scaling1 : Subsystem
  Divide1 : Product  Inputs=*/
  Gain : Gain  Gain=2
  Mass Diffusion Coeffecient [m^2 /s]1 : Subsystem
  Math Function : Math  Operator=pow  SaturateOnIntegerOverflow=on
  Math Function1 : Math  Operator=pow  SaturateOnIntegerOverflow=on
  Product : Product
  Re_Num  Scaled : Subsystem
  Schmidt Number : Subsystem
  Sherwood Number : Product  Inputs=4
  Viscosity W Scaling1 : Subsystem
  k_m_b : Outport
  wires:
  Constant1/1 -> Math Function/2
  [r_b] -> Gain/1
  Constant2/1 -> Math Function1/2
  [D_FS_Local] -> Divide1/1
  Constant4/1 -> Sherwood Number/3
  Constant/1 -> Sherwood Number/1
  Divide1/1 -> Product/2
  Math Function1/1 -> Sherwood Number/4
  Schmidt Number/1(Sc) -> Math Function1/1
  Math Function/1 -> Sherwood Number/2
  Sherwood Number/1 -> Product/1
  Product/1 -> k_m_b/1
  Re_Num  Scaled/1(Re) -> Math Function/1
  [Mu_FS_Local] -> Schmidt Number/1(mu)
  [Rho_FS_Local] -> Schmidt Number/2(rho)
  [D_FS_Local] -> Schmidt Number/3(D)
  T/1 -> Mass Diffusion Coeffecient [m^2 /s]1/2(T_Salt [k]), Viscosity W Scaling1/1(T_Salt [k]), Density W Scaling1/1(T_Salt [k]), Re_Num  Scaled/1(T)
  Density W Scaling1/1(rho_FS [kg/m^3]) -> [Rho_FS_Local]
  Viscosity W Scaling1/1(mu [Pa-s]) -> Mass Diffusion Coeffecient [m^2 /s]1/1(Mu), [Mu_FS_Local]
  Mass Diffusion Coeffecient [m^2 /s]1/1(D [m^2/s]) -> [D_FS_Local]
  Constant3/1 -> Re_Num  Scaled/2(Re_0)
  Gain/1 -> Divide1/2

== system Xe_Model_Redo_June_26/Bubbles/Bubble Mass Transfer/P100/HRT*C_B /Calc H_Xe ==
  T_Salt [K] : Inport
  Constant : Constant  Value=H_Xe_c
  Math Function : Math  Operator=magnitude^2  SaturateOnIntegerOverflow=on
  Sum1 : Sum  Inputs=+++
  a const : Gain  Gain=H_Xe_a
  b const : Gain  Gain=H_Xe_b
  H_Xe [m^-3 Pa^-1] : Outport
  wires:
  Sum1/1 -> H_Xe [m^-3 Pa^-1]/1
  a const/1 -> Sum1/1
  Constant/1 -> Sum1/3
  b const/1 -> Sum1/2
  Math Function/1 -> a const/1
  T_Salt [K]/1 -> b const/1, Math Function/1

== system Xe_Model_Redo_June_26/Bubbles/Bubble Mass Transfer/P100/KMA_P100/CA  CV Area ==
  Node Vol. : Inport
  CV Vol to Mass Transfer Area1 : Subsystem
  A : Outport
  wires:
  CV Vol to Mass Transfer Area1/1(A) -> A/1
  Node Vol./1 -> CV Vol to Mass Transfer Area1/1(V)
